simulink model "positive_solution"  (R2023b)
settings: Solver=ode4  StartTime=0.0  StopTime=20  FixedStep=0.0001  MaxStep=2e-4  RelTol=1e-3
libraries: sm_lib x5
settings Model: Creator=ZLX  LastModifiedBy=ZLX

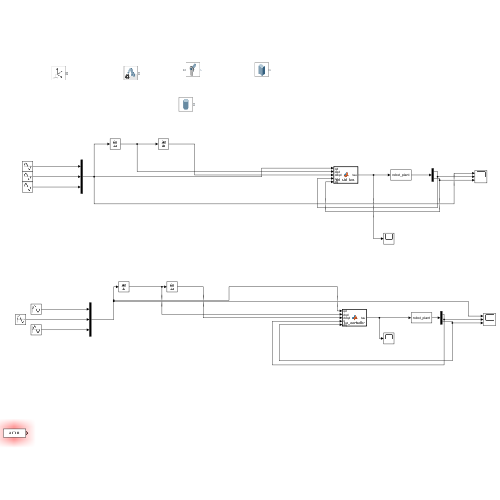
[thumbnail: Simulink's stored preview of the top-level diagram]
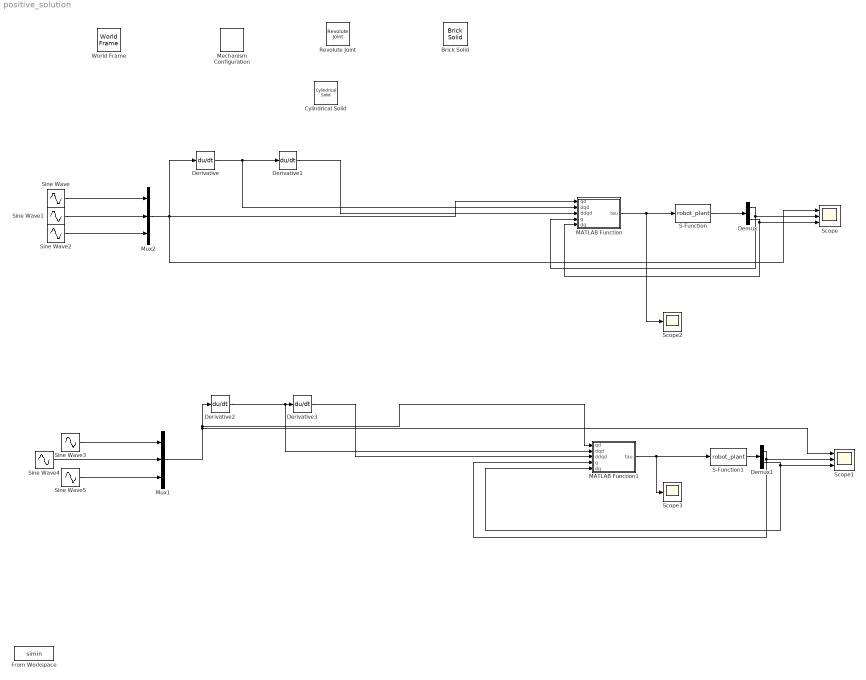
== system positive_solution ==
  Brick Solid : sm_lib/Body Elements/Brick Solid  GraphicAmbientColor=[0.15 0.15 0.15 1.0]  BasedOnType=Density  BrickDimensions=[1 1 1]  BrickDimensionsUnits=m  CenterOfMass=[0 0 0]  CenterOfMassUnits=m  GraphicDiffuseColor=[0.5 0.5 0.5]  Density=1000  DensityUnits=kg/m^3  DoExposeReferenceFrame=on  GraphicEmissiveColor=[0.0 0.0 0.0 1.0]  ExportEntireGeometry=off  SerializedFrames=<Frames/>  MarkerShape=Sphere  MarkerSize=10  GraphicType=FromGeometry  InertiaType=CalculateFromGeometry  Mass=1  MassUnits=kg  MomentsOfInertia=[1 1 1]  MomentsOfInertiaUnits=kg*m^2  GraphicOpacity=1.0  ProductsOfInertia=[0 0 0]  ProductsOfInertiaUnits=kg*m^2  GraphicShininess=75  GraphicSpecularColor=[0.5 0.5 0.5 1.0]  GraphicVisPropType=SimpleVisualProperties
  Cylindrical Solid : sm_lib/Body Elements/Cylindrical Solid  GraphicAmbientColor=[0.15 0.15 0.15 1.0]  BasedOnType=Density  CenterOfMass=[0 0 0]  CenterOfMassUnits=m  GraphicDiffuseColor=[0.5 0.5 0.5]  CylinderLength=1  CylinderLengthUnits=m  CylinderRadius=1  CylinderRadiusUnits=m  Density=1000  DensityUnits=kg/m^3  DoExposeReferenceFrame=on  GraphicEmissiveColor=[0.0 0.0 0.0 1.0]  ExportEntireGeometry=off  SerializedFrames=<Frames/>  MarkerShape=Sphere  MarkerSize=10  GraphicType=FromGeometry  InertiaType=CalculateFromGeometry  Mass=1  MassUnits=kg  MomentsOfInertia=[1 1 1]  MomentsOfInertiaUnits=kg*m^2  GraphicOpacity=1.0  ProductsOfInertia=[0 0 0]  ProductsOfInertiaUnits=kg*m^2  GraphicShininess=75  GraphicSpecularColor=[0.5 0.5 0.5 1.0]  GraphicVisPropType=SimpleVisualProperties
  Demux : Demux  Outputs=[3 3]
  Demux1 : Demux  Outputs=[3 3]
  Derivative{,1..3} (4 alike) : Derivative
  From Workspace : FromWorkspace  VariableName=simin
  MATLAB Function : MATLAB Function  TreatAsAtomicUnit=on
  MATLAB Function1 : MATLAB Function  TreatAsAtomicUnit=on
  Mechanism Configuration : sm_lib/Utilities/Mechanism Configuration  UniformGravity=Constant  GravityVector=[0 0 -9.80665]  GravityVectorUnits=m/s^2  LinearizationDelta=0.001  JointModeTransitionNonlinearIterations=2
  Mux1 : Mux  Inputs=3
  Mux2 : Mux  Inputs=3
  Revolute Joint : sm_lib/Joints/Revolute Joint  JointMode=Normal  SenseConstraintForce=off  SenseConstraintForceX=off  SenseConstraintForceY=off  SenseConstraintForceZ=off  SenseConstraintTorque=off  SenseConstraintTorqueX=off  SenseConstraintTorqueY=off  SenseConstraintTorqueZ=off  SenseTotalForce=off  SenseTotalForceX=off  SenseTotalForceY=off  SenseTotalForceZ=off  SenseTotalTorque=off  SenseTotalTorqueX=off  SenseTotalTorqueY=off  SenseTotalTorqueZ=off  CompositeWrenchDir=FollowerOnBase  CompositeWrenchFrame=BaseFrame  EquilibriumPosition=0  EquilibriumPositionUnits=deg  SpringStiffness=0  SpringStiffnessUnits=N*m/deg  DampingCoefficient=0  DampingCoefficientUnits=N*m/(deg/s)  TorqueActuationMode=NoTorque  MotionActuationMode=ComputedMotion  SensePosition=off  SenseVelocity=off  SenseAcceleration=off  SenseTorqueForce=off  SenseLowerLimitTorqueForce=off  SenseUpperLimitTorqueForce=off  LowerLimitSpecify=off  LowerLimitBound=-90  LowerLimitBoundUnits=deg  LowerLimitStiffness=1e4  LowerLimitStiffnessUnits=N*m/deg  LowerLimitDamping=10  LowerLimitDampingUnits=N*m/(deg/s)  LowerLimitTransitionRegionWidth=0.1  LowerLimitTransitionRegionWidthUnits=deg  UpperLimitSpecify=off  UpperLimitBound=90  UpperLimitBoundUnits=deg  UpperLimitStiffness=1e4  UpperLimitStiffnessUnits=N*m/deg  UpperLimitDamping=10  UpperLimitDampingUnits=N*m/(deg/s)  UpperLimitTransitionRegionWidth=0.1  UpperLimitTransitionRegionWidthUnits=deg  PositionTargetSpecify=off  PositionTargetPriority=High  PositionTargetValue=0  PositionTargetValueUnits=deg  VelocityTargetSpecify=off  VelocityTargetPriority=High  VelocityTargetValue=0  VelocityTargetValueUnits=deg/s
  S-Function : S-Function  FunctionName=robot_plant  SFunctionDeploymentMode=off  EnableBusSupport=off
  S-Function1 : S-Function  FunctionName=robot_plant  SFunctionDeploymentMode=off  EnableBusSupport=off
  Scope : Scope  NumInputPorts=3
  Scope1 : Scope  NumInputPorts=3
  Scope2 : Scope
  Scope3 : Scope
  Sine Wave : Sin  Frequency=2  SampleTime=0
  Sine Wave1 : Sin  Frequency=2  Phase=0.15  SampleTime=0
  Sine Wave2 : Sin  Frequency=2  Phase=0.3  SampleTime=0
  Sine Wave3 : Sin  Frequency=2  SampleTime=0
  Sine Wave4 : Sin  Frequency=2  Phase=0.15  SampleTime=0
  Sine Wave5 : Sin  Frequency=2  Phase=0.3  SampleTime=0
  World Frame : sm_lib/Frames and Transforms/World Frame
  wires:
  S-Function/1 -> Demux/1
  Demux/1 -> MATLAB Function/4(q), Scope/2
  Demux/2 -> MATLAB Function/5(dq), Scope/3
  Mux2/1 -> MATLAB Function/1(qd), Derivative/1, Scope/1
  Derivative/1 -> MATLAB Function/2(dqd), Derivative1/1
  Sine Wave/1 -> Mux2/1
  Sine Wave1/1 -> Mux2/2
  Sine Wave2/1 -> Mux2/3
  Derivative1/1 -> MATLAB Function/3(ddqd)
  MATLAB Function/1(tau) -> Scope2/1, S-Function/1
  MATLAB Function1/1(tau) -> Scope3/1, S-Function1/1
  Derivative3/1 -> MATLAB Function1/3(ddqd)
  Sine Wave5/1 -> Mux1/3
  Demux1/1 -> MATLAB Function1/4(q), Scope1/2
  Sine Wave3/1 -> Mux1/1
  Derivative2/1 -> MATLAB Function1/2(dqd), Derivative3/1
  Mux1/1 -> Scope1/1, MATLAB Function1/1(qd), Derivative2/1
  Sine Wave4/1 -> Mux1/2
  Demux1/2 -> MATLAB Function1/5(dq), Scope1/3
  S-Function1/1 -> Demux1/1

== matlab function positive_solution/MATLAB Function1 ==
  settings: updateMethod=DISCRETE
  data: qd input; tau output; dqd input; ddqd input; q input; dq input
function tau = pid_controller(qd, dqd, ddqd, q, dq)
% PID Controller for Comparison
% 输入接口保持与 RBF 控制器一致，方便直接替换

% --- 1. 定义状态变量 ---
persistent error_sum
if isempty(error_sum)
    error_sum = zeros(3,1); % 积分项累加器
end

% --- 2. PID 参数整定 (经验值) ---
% 这里的参数需要调得比较大才能跟上 RBF 的效果
% 针对关节 1 (基座), 2 (肩), 3 (肘) 分别设置
Kp = diag([500, 500, 500]);  % 比例增益：决定“力气”有多大
Ki = diag([200, 200, 200]);  % 积分增益：消除静差 (抵抗重力)
Kd = diag([20, 20, 20]);     % 微分增益：提供阻尼 (防止震荡)

% --- 3. 计算误差 ---
e = qd - q;       % 位置误差
de = dqd - dq;    % 速度误差

% --- 4. 积分计算 (抗饱和) ---
dt = 0.0001; % 必须与 Simulink Solver 步长一致！(如果你是 0.0001 请修改这里)
error_sum = error_sum + e * dt;

% 积分限幅 (Anti-windup)：防止误差累积过大导致超调
limit_I = 20; 
error_sum = max(min(error_sum, limit_I), -limit_I);

% --- 5. 计算输出力矩 ---
% 标准 PID 公式: tau = Kp*e + Ki*sum + Kd*de
tau = Kp*e + Ki*error_sum + Kd*de;

% --- 6. 输出限幅 ---
tau = max(min(tau, 1000), -1000); % 与 RBF 保持一致的物理限制

end

== matlab function positive_solution/MATLAB Function ==
  settings: updateMethod=DISCRETE
  data: qd input; tau output; dqd input; ddqd input; q input; dq input
function tau = rbf_ctrl_fast(qd, dqd, ddqd, q, dq)
% MATLAB Function: 高性能 RBF-SMC 控制器
% 配置: Lambda=25, Gamma=50, Kv=20, dt=0.1ms

% --- 1. 参数定义 ---
persistent W_hat 
persistent Centers

% 初始化
if isempty(W_hat)
    W_hat = zeros(30, 1); 
    
    % 【优化建议】扩大 RBF 中心的覆盖范围
    % 既然 Lambda=25，误差 s 的变化范围可能会变大
    % 将中心范围从 [-2.5, 2.5] 扩大一点，或者保持不变
    Centers = zeros(6, 10);
    for j = 1:10
        Centers(:,j) = (j - 10/2) * 0.5; 
    end
end

% --- 2. 误差计算 ---
e = qd - q;
de = dqd - dq;
% 高增益: 加快收敛速度，但需注意噪声放大
Lambda = diag([40, 40, 40]); 
s = de + Lambda * e;

% --- 3. RBF 激活 ---
Z = [e; de]; 
B_width = 1.0;
h = zeros(10, 1);

for j = 1:10
    dist = norm(Z - Centers(:,j))^2;
    h(j) = exp(-dist / (2 * B_width^2));
end

% --- 4. 权重自适应更新 ---
Gamma = 100; % 高学习率

W_matrix = reshape(W_hat, 10, 3);

% 【死区检查】
% 0.002 非常小。如果发现权重漂移，可以稍微放宽到 0.005
if norm(s) < 0.002
    dW_matrix = zeros(10, 3);
else
    dW_matrix = Gamma * (h * s');
end

% 离散积分
% ⚠️ 务必确保 Simulink Solver Fixed-step size = 0.0001
dt = 0.0001; 
W_matrix = W_matrix + dW_matrix * dt;

W_hat = W_matrix(:);

% --- 5. 控制输出 ---
f_hat = W_matrix' * h; 

% 高鲁棒增益: 压制未建模误差
Kv = diag([20, 20, 20]); 

M_approx = diag([2.0, 1.5, 1.0]); 
dqr = dqd + Lambda * e;
ddqr = ddqd + Lambda * de;

tau = M_approx * ddqr + Kv * s + f_hat; 

% 限幅
tau = max(min(tau, 1000), -1000);

end
